simulink model "HQEV_MiL_20160830_integrate"  (Simulink 8.3)
settings: Solver=FixedStepDiscrete  StartTime=0.0  StopTime=inf  FixedStep=0.01  RelTol=1e-3
PostLoadFcn:
  | , if any(exist('dsrtsu_mdlpostloadfcn', 'file') == [2, 3, 6]), try dsrtsu_mdlpostloadfcn('Execute', bdroot); catch fprintf('Error in PostLoadFcn (dsrtsu_mdlpostloadfcn) for model "%s":\n %s\n', bdroot, lasterr); end, end,
values from neighbouring files (symbols this model uses):
  Bat_C_Ah = 36    [parameter_V1.mat]
  Bat_ocv_xIndex = [5 10 20 30 40 50 60 70 80 90 95]    [parameter_V1.mat]
  Bat_ocv_z = [329 332 340 345 347 351 358 372 377 386 391]    [parameter_V1.mat]
  Bat_R_ohm_z = [4.41 3.46 1.57 1.07 0.76 0.63 0.55 0.44 0.41 0.4 0.4 3.14 ... (66 elements, 11x6)]    [parameter_V1.mat]
  Bat_SOC_Init = 90    [parameter_V1.mat]
  Env_hum_pct_Ambient = 30    [parameter_V1.mat]
  Env_Slope_deg = 0    [parameter_V1.mat]
  Env_Temp_degC_Ambient = 25    [parameter_V1.mat]
  Env_v_kmph_HWind = 0    [parameter_V1.mat]
  Reducer_F_i = 7.23    [parameter_V1.mat]
  Reducer_R_i = 7.23    [parameter_V1.mat]
  Veh =     [parameter_V1.mat]
  Veh_A_m2_Fr = 2.246    [parameter_V1.mat]
  Veh_F_Brake =     [parameter_V1.mat]
  Veh_fac_AirDrag = 0.326    [parameter_V1.mat]
  Veh_fac_WhDragFrict_0 = 0.011    [parameter_V1.mat]
  Veh_g_mps2_C = 9.81    [parameter_V1.mat]
  Veh_GainBrake =     [parameter_V1.mat]
  Veh_h_m_COGHigh = 0.5    [parameter_V1.mat]
  Veh_J_kgm2_Wh = 1.3635    [parameter_V1.mat]
  Veh_L_m_AxlBas = 2.63    [parameter_V1.mat]
  Veh_M_kg = 1427    [parameter_V1.mat]
  Veh_mu_Brake = 0.4    [parameter_V1.mat]
  Veh_mu_Tyre =     [parameter_V1.mat]
  Veh_num_FrictPair = 8    [parameter_V1.mat]
  Veh_pct_Brk = 70    [parameter_V1.mat]
  Veh_r_dyn =     [parameter_V1.mat]
  Veh_r_m_BrkDisk = 0.136    [parameter_V1.mat]
  Veh_rho_kgpm3_Air = 1.2258    [parameter_V1.mat]
undefined symbols (not defined in the file or in its folder): DiscIntNeverNeededParam, p_bool_False_M, p_bool_True_M
libraries: BaseOperationLib_Browser x38, simulink x9, DTQC_lib x1, ERR_lib x1, MQM_lib x1, PTCL_lib x1, PUD_lib x1, TQD_lib x1, TQR_lib x1, VMM_lib x1, ACCA_lib x1, BBCA_lib x1
(part 13 of 15)

== system HQEV_MiL_20160830_integrate/MiL/Test_Integration/Charger/Charger/Charger/Charger/Abnormal/Subsystem ==
  Constant2 : Constant  Value=3
  Constant3 : Constant  Value=0
  Constant4 : Constant  Value=0
  Constant5 : Constant  Value=0
  Constant6 : Constant  Value=30
  ChargerOutputVoltage : Outport
  ChargerOutputCurrent : Outport  Port=2
  ChargerStatus : Outport  Port=3
  RechargeRequest : Outport  Port=4
  ChargerTemperature : Outport  Port=5
  wires:
  Constant2/1 -> ChargerStatus/1
  Constant5/1 -> RechargeRequest/1
  Constant6/1 -> ChargerTemperature/1
  Constant3/1 -> ChargerOutputVoltage/1
  Constant4/1 -> ChargerOutputCurrent/1

== system HQEV_MiL_20160830_integrate/MiL/Test_Integration/Charger/Charger/Charger/Charger/Fault/Subsystem ==
  Constant2 : Constant  Value=3
  Constant3 : Constant  Value=0
  Constant4 : Constant  Value=0
  Constant5 : Constant  Value=0
  Constant6 : Constant  Value=30
  ChargerOutputVoltage : Outport
  ChargerOutputCurrent : Outport  Port=2
  ChargerStatus : Outport  Port=3
  RechargeRequest : Outport  Port=4
  ChargerTemperature : Outport  Port=5
  wires:
  Constant2/1 -> ChargerStatus/1
  Constant5/1 -> RechargeRequest/1
  Constant6/1 -> ChargerTemperature/1
  Constant3/1 -> ChargerOutputVoltage/1
  Constant4/1 -> ChargerOutputCurrent/1

== system HQEV_MiL_20160830_integrate/MiL/Test_Integration/Charger/Charger/Charger/Charger/Idle/Subsystem ==
  CC : Inport
  ACChargeStation_U : Inport  Port=2
  Chart : Stateflow chart  TreatAsAtomicUnit=on
  Constant : Constant  Value=200
  Constant1 : Constant  Value=0
  Constant2 : Constant  Value=0
  Constant3 : Constant  Value=0
  Constant4 : Constant  Value=30
  Logical Operator : Logic  Operator=NOT  AllPortsSameDT=off  OutDataTypeStr=boolean
  Relational Operator : RelationalOperator  OutDataTypeStr=boolean
  ChargerOutputVoltage : Outport
  ChargerOutputCurrent : Outport  Port=2
  ChargerStatus : Outport  Port=3
  RechargeRequest : Outport  Port=4
  ChargerTemperature : Outport  Port=5
  wires:
  ACChargeStation_U/1 -> Relational Operator/1
  Constant/1 -> Relational Operator/2
  Relational Operator/1 -> Chart/1(PowerOn), Logical Operator/1
  Logical Operator/1 -> Chart/2(PowerOff)
  CC/1 -> Chart/3(CC)
  Chart/1(RechargeRequest) -> RechargeRequest/1
  Constant1/1 -> ChargerOutputVoltage/1
  Constant2/1 -> ChargerStatus/1
  Constant3/1 -> ChargerOutputCurrent/1
  Constant4/1 -> ChargerTemperature/1

== system HQEV_MiL_20160830_integrate/MiL/Test_Integration/Charger/Charger/Charger/Charger/Work/Subsystem ==
  HCU_ChargePermission : Inport
  BMS_MainPosContactorState : Inport  Port=2
  HCU_ChargeHeatingPermission : Inport  Port=3
  BMS_MainNegContactorState : Inport  Port=4
  BMS_PreChargeContactorState : Inport  Port=5
  BMS_ChargePosContactorState : Inport  Port=6
  BMS_ChargeNegContactorState : Inport  Port=7
  AC_Charge : Subsystem  TreatAsAtomicUnit=on
  Constant : Subsystem
  ChargerOutputVoltage : Outport
  ChargerOutputCurrent : Outport  Port=2
  ChargerStatus : Outport  Port=3
  RechargeRequest : Outport  Port=4
  ChargerTemperature : Outport  Port=5
  wires:
  AC_Charge/1(ChargerOutputVoltage) -> ChargerOutputVoltage/1
  AC_Charge/2(ChargerOutputCurrent) -> ChargerOutputCurrent/1
  Constant/1(ChargerStatus) -> ChargerStatus/1
  Constant/2(RechargeRequest) -> RechargeRequest/1
  Constant/3(ChargerTemperature) -> ChargerTemperature/1
  HCU_ChargePermission/1 -> AC_Charge/1(HCU_ChargePermission)
  BMS_MainPosContactorState/1 -> AC_Charge/2(BMS_MainPosContactorState)
  HCU_ChargeHeatingPermission/1 -> AC_Charge/3(HCU_ChargeHeatingPermission)
  BMS_MainNegContactorState/1 -> AC_Charge/4(BMS_MainNegContactorState)
  BMS_PreChargeContactorState/1 -> AC_Charge/5(BMS_PreChargeContactorState)
  BMS_ChargePosContactorState/1 -> AC_Charge/6(BMS_ChargePosContactorState)
  BMS_ChargeNegContactorState/1 -> AC_Charge/7(BMS_ChargeNegContactorState)

== system HQEV_MiL_20160830_integrate/MiL/Test_Integration/Driver/Driver/Driver_AutoPedal/CTRL AccPed/Reset/Compare To Constant ==
  u : Inport
  Compare : RelationalOperator  Operator=<  OutDataTypeStr=boolean  ZeroCross=off  InputSameDT=on
  Constant : Constant  Value=const  OutDataTypeStr=Inherit: Inherit via back propagation
  y : Outport
  wires:
  u/1 -> Compare/1
  Constant/1 -> Compare/2
  Compare/1 -> y/1

== system HQEV_MiL_20160830_integrate/MiL/Test_Integration/Driver/Driver/Driver_AutoPedal/CTRL AccPed/Reset/Compare To Constant1 ==
  u : Inport
  Compare : RelationalOperator  Operator=>  OutDataTypeStr=boolean  ZeroCross=off  InputSameDT=on
  Constant : Constant  Value=const  OutDataTypeStr=Inherit: Inherit via back propagation
  y : Outport
  wires:
  u/1 -> Compare/1
  Constant/1 -> Compare/2
  Compare/1 -> y/1

== system HQEV_MiL_20160830_integrate/MiL/Test_Integration/Driver/Driver/Driver_AutoPedal/CTRL AccPed/Reset/v_Set==0  ==
  u : Inport
  Compare : RelationalOperator  Operator=<=  OutDataTypeStr=uint(8)  ZeroCross=off  InputSameDT=on
  Constant : Constant  Value=const  OutDataTypeStr=Inherit: Inherit via back propagation
  y : Outport
  wires:
  u/1 -> Compare/1
  Constant/1 -> Compare/2
  Compare/1 -> y/1

== system HQEV_MiL_20160830_integrate/MiL/Test_Integration/Driver/Driver/Driver_AutoPedal/CTRL BrakePed/Reset_Block/Compare To Constant2 ==
  u : Inport
  Compare : RelationalOperator  Operator=>  OutDataTypeStr=uint(8)  ZeroCross=off  InputSameDT=on
  Constant : Constant  Value=const  OutDataTypeStr=Inherit: Inherit via back propagation
  y : Outport
  wires:
  Compare/1 -> y/1
  Constant/1 -> Compare/2
  u/1 -> Compare/1

== system HQEV_MiL_20160830_integrate/MiL/Test_Integration/Driver/Driver/Driver_AutoPedal/CTRL BrakePed/Reset_Block/Compare To Constant7 ==
  u : Inport
  Compare : RelationalOperator  Operator===  OutDataTypeStr=uint(8)  ZeroCross=off  InputSameDT=on
  Constant : Constant  Value=const  OutDataTypeStr=Inherit: Inherit via back propagation
  y : Outport
  wires:
  Compare/1 -> y/1
  Constant/1 -> Compare/2
  u/1 -> Compare/1

== system HQEV_MiL_20160830_integrate/MiL/Test_Integration/Driver/Driver/Driver_AutoPedal/CTRL BrakePed/Set_Block/Compare To Constant1 ==
  u : Inport
  Compare : RelationalOperator  Operator=<  OutDataTypeStr=boolean  ZeroCross=off  InputSameDT=on
  Constant : Constant  Value=const  OutDataTypeStr=Inherit: Inherit via back propagation
  y : Outport
  wires:
  Compare/1 -> y/1
  Constant/1 -> Compare/2
  u/1 -> Compare/1

== system HQEV_MiL_20160830_integrate/MiL/Test_Integration/Driver/Driver/Driver_AutoPedal/CTRL BrakePed/Set_Block/Compare To Constant3 ==
  u : Inport
  Compare : RelationalOperator  Operator=>  OutDataTypeStr=boolean  ZeroCross=off  InputSameDT=on
  Constant : Constant  Value=const  OutDataTypeStr=Inherit: Inherit via back propagation
  y : Outport
  wires:
  Compare/1 -> y/1
  Constant/1 -> Compare/2
  u/1 -> Compare/1

== system HQEV_MiL_20160830_integrate/MiL/Test_Integration/Driver/Driver/Driver_AutoPedal/CTRL BrakePed/Set_Block/Compare To Constant5 ==
  u : Inport
  Compare : RelationalOperator  Operator===  OutDataTypeStr=boolean  ZeroCross=off  InputSameDT=on
  Constant : Constant  Value=const  OutDataTypeStr=Inherit: Inherit via back propagation
  y : Outport
  wires:
  Compare/1 -> y/1
  Constant/1 -> Compare/2
  u/1 -> Compare/1

== system HQEV_MiL_20160830_integrate/MiL/Test_Integration/Driver/Driver/Driver_AutoPedal/CTRL BrakePed/Set_Block/Compare To Constant6 ==
  u : Inport
  Compare : RelationalOperator  Operator=>  OutDataTypeStr=boolean  ZeroCross=off  InputSameDT=on
  Constant : Constant  Value=const  OutDataTypeStr=Inherit: Inherit via back propagation
  y : Outport
  wires:
  Compare/1 -> y/1
  Constant/1 -> Compare/2
  u/1 -> Compare/1

== system HQEV_MiL_20160830_integrate/MiL/Test_Integration/Driver/Driver/Driver_AutoPedal/CTRL BrakePed/velocoty/Run_Forward ==
  v_set : Inport
  v_Veh : Inport  Port=2
  Difference : Subsystem
      mask Display: disp('')
  Gain1 : Gain  Gain=-1
  Subtract : Sum  Inputs=+-
  delta_v_set : Outport
  error : Outport  Port=2
  wires:
  v_set/1 -> Difference/1(In1), Subtract/1
  v_Veh/1 -> Subtract/2
  Difference/1(Out1) -> delta_v_set/1
  Subtract/1 -> Gain1/1
  Gain1/1 -> error/1

== system HQEV_MiL_20160830_integrate/MiL/Test_Integration/HCU/HCU/HCU/EVManager/evm_core/DTQC ==
  Bus_TQD : Inport
  Bus_hw_prep : Inport  Port=2
  Bus_hw_algo : Inport  Port=3
  Bus_PTC1 : BusSelector  OutputSignals=pTQD_Nm_MCU1TMTorqReq,pTQD_Nm_MCU2TMTorqReq
  Bus_PTC2 : BusSelector  OutputSignals=Bus_ESPI.pESPI_bool_ABSIntv,Bus_ESPI.pESPI_Nm_ABS1IntvTrqReq,Bus_ESPI.pESPI_Nm_ABS2IntvTrqReq,Bus_ESPI.pESPI_bool_ASR1Intv,Bus_ESPI.pESPI_Nm_ASR1IntvTrqReq,Bus_ESPI.pESPI_bool_ASR2Intv,Bus_ESPI.pESPI_Nm_ASR2IntvTrqReq,Bus_ESPI.pESPI_bool_RBSIntv,Bus_ESPI.pESPI_Nm_RBSIntvTrqReq,Bus_ESPI.pESPI_bool_MSR1Intv,Bus_ESPI.pESPI_Nm_MSR1IntvTrqReq,Bus_ESPI.pESPI_bool_MSR2Intv,Bus_ESPI.pESPI_Nm_MSR2IntvTrqReq
  Bus_PTC3 : BusSelector  OutputSignals=Bus_ACCI.pACCI_bool_AEBIntv,Bus_ACCI.pACCI_Nm_AEBTM1TrqReq,Bus_ACCI.pACCI_Nm_AEBTM2TrqReq
  Bus_TQD_out : BusCreator  Inputs=3
  DTQC : DTQC_lib/DTQC  SystemSampleTime=-1
  Terminator : Terminator
  Bus_DTQC : Outport
  wires:
  Bus_PTC3/3 -> DTQC/18  "<pACCI_Nm_AEBTM2TrqReq>"
  Bus_PTC3/2 -> DTQC/17  "<pACCI_Nm_AEBTM1TrqReq>"
  Bus_PTC3/1 -> DTQC/16  "<pACCI_bool_AEBIntv>"
  Bus_hw_algo/1 -> Terminator/1
  Bus_PTC2/13 -> DTQC/13  "<pESPI_Nm_MSR2IntvTrqReq>"
  Bus_PTC2/12 -> DTQC/12  "<pESPI_bool_MSR2Intv>"
  Bus_PTC2/11 -> DTQC/11  "<pESPI_Nm_MSR1IntvTrqReq>"
  Bus_PTC2/10 -> DTQC/10  "<pESPI_bool_MSR1Intv>"
  Bus_PTC2/9 -> DTQC/9  "<pESPI_Nm_RBSIntvTrqReq>"
  Bus_PTC2/8 -> DTQC/8  "<pESPI_bool_RBSIntv>"
  Bus_PTC2/7 -> DTQC/7  "<pESPI_Nm_ASR2IntvTrqReq>"
  Bus_PTC2/6 -> DTQC/6  "<pESPI_bool_ASR2Intv>"
  Bus_PTC2/5 -> DTQC/5  "<pESPI_Nm_ASR1IntvTrqReq>"
  Bus_PTC2/4 -> DTQC/4  "<pESPI_bool_ASR1Intv>"
  Bus_PTC2/3 -> DTQC/3  "<pESPI_Nm_ABS2IntvTrqReq>"
  Bus_PTC2/2 -> DTQC/2  "<pESPI_Nm_ABS1IntvTrqReq>"
  Bus_PTC2/1 -> DTQC/1  "<pESPI_bool_ABSIntv>"
  Bus_hw_prep/1 -> Bus_PTC3/1, Bus_PTC2/1
  Bus_PTC1/2 -> DTQC/15  "<pTQD_Nm_MCU2TMTorqReq>"
  Bus_PTC1/1 -> DTQC/14  "<pTQD_Nm_MCU1TMTorqReq>"
  DTQC/3 -> Bus_TQD_out/3
  DTQC/2 -> Bus_TQD_out/2
  DTQC/1 -> Bus_TQD_out/1
  Bus_TQD/1 -> Bus_PTC1/1
  Bus_TQD_out/1 -> Bus_DTQC/1  "Bus_DTQC"

== system HQEV_MiL_20160830_integrate/MiL/Test_Integration/HCU/HCU/HCU/EVManager/evm_core/ERR ==
  Bus_hw_prep : Inport
  Bus_hw_algo : Inport  Port=2
  Bus Selector : BusSelector  OutputSignals=Bus_ARBI.pARBI_st_StCrash,Bus_MCI.pMCI_st_MotCtrlErr,Bus_TBCI.pTBCI_st_ChrgrErr,Bus_BMSI.pBMSI_st_BMSErr,Bus_SHLI.pSHLI_st_ShftLvrErr,Bus_ESPI.pESPI_kmph_VehLgtSpd
  Bus Selector1 : BusSelector  OutputSignals=Bus_SHLA.pSHLA_st_PrkgLockFlt
  Bus Selector2 : BusSelector  OutputSignals=Bus_BRPI.pBRPI_st_BrkPedErr,Bus_ARBI.pARBI_st_AirBagErr,Bus_EPSI.pEPSI_st_EPSErr,Bus_DCCI.pDCCI_st_DCDCErr,Bus_TMCI.pTMCI_bool_AirCdnErr,Bus_TMCI.pTMCI_st_AC1PTCSt
  Bus Selector4 : BusSelector  OutputSignals=Bus_TBCI.pTBCI_st_ChrgrPlgTempErr,Bus_BMSI.pBMSI_st_DCChrgrErr
  ERR : ERR_lib/ERR  SystemSampleTime=-1
  err_bb : BusCreator  Inputs=2
  Bus_ERR : Outport
  wires:
  Bus Selector/6 -> ERR/6  "<pESPI_kmph_VehLgtSpd>"
  ERR/2 -> err_bb/2
  Bus Selector2/2 -> ERR/9  "<pARBI_st_AirBagErr>"
  Bus Selector2/1 -> ERR/8  "<pBRPI_st_BrkPedErr>"
  Bus Selector4/2 -> ERR/15  "<pBMSI_st_DCChrgrErr>"
  Bus Selector4/1 -> ERR/14  "<pTBCI_st_ChrgrPlgTempErr>"
  Bus Selector2/5 -> ERR/12  "<pTMCI_bool_AirCdnErr>"
  Bus Selector2/4 -> ERR/11  "<pDCCI_st_DCDCErr>"
  Bus Selector2/3 -> ERR/10  "<pEPSI_st_EPSErr>"
  Bus Selector1/1 -> ERR/7  "<pSHLA_st_PrkgLockFlt>"
  Bus_hw_algo/1 -> Bus Selector1/1
  Bus Selector/5 -> ERR/5  "<pSHLI_st_ShftLvrErr>"
  Bus Selector/4 -> ERR/4  "<pBMSI_st_BMSErr>"
  Bus Selector/3 -> ERR/3  "<pTBCI_st_ChrgrErr>"
  Bus Selector/2 -> ERR/2  "<pMCI_st_MotCtrlErr>"
  Bus Selector/1 -> ERR/1  "<pARBI_st_StCrash>"
  ERR/1 -> err_bb/1
  err_bb/1 -> Bus_ERR/1  "Bus_ERR"
  Bus_hw_prep/1 -> Bus Selector/1, Bus Selector4/1, Bus Selector2/1
  Bus Selector2/6 -> ERR/13  "<pTMCI_st_AC1PTCSt>"

== system HQEV_MiL_20160830_integrate/MiL/Test_Integration/HCU/HCU/HCU/EVManager/evm_core/MQM ==
  Bus_DTQC : Inport
  Bus_hw_prep : Inport  Port=2
  Bus_hw_algo : Inport  Port=3
  Bus_PTC1 : BusSelector  OutputSignals=pDTQC_Nm_MCU1TMTorqReq,pDTQC_Nm_MCU2TMTorqReq
  Bus_PTC2 : BusSelector  OutputSignals=Bus_MCI.pMCI_Nm_MCU1MotCtrlActTrq,Bus_MCI.pMCI_Nm_MCU2MotCtrlActTrq
  Bus_PTC3 : BusSelector  OutputSignals=Bus_SHLA.pSHLA_st_ShiftLvrPosn
  Bus_TQD_out : BusCreator  Inputs=3
  MQM : MQM_lib/MQM  SystemSampleTime=-1
  Bus_MQM : Outport
  wires:
  Bus_PTC3/1 -> MQM/5  "<pSHLA_st_ShiftLvrPosn>"
  Bus_hw_algo/1 -> Bus_PTC3/1
  Bus_PTC2/2 -> MQM/4  "<pMCI_Nm_MCU2MotCtrlActTrq>"
  Bus_PTC2/1 -> MQM/3  "<pMCI_Nm_MCU1MotCtrlActTrq>"
  Bus_hw_prep/1 -> Bus_PTC2/1
  Bus_PTC1/2 -> MQM/2  "<pDTQC_Nm_MCU2TMTorqReq>"
  Bus_PTC1/1 -> MQM/1  "<pDTQC_Nm_MCU1TMTorqReq>"
  Bus_TQD_out/1 -> Bus_MQM/1  "Bus_MQM"
  Bus_DTQC/1 -> Bus_PTC1/1
  MQM/1 -> Bus_TQD_out/1
  MQM/2 -> Bus_TQD_out/2
  MQM/3 -> Bus_TQD_out/3

== system HQEV_MiL_20160830_integrate/MiL/Test_Integration/HCU/HCU/HCU/EVManager/evm_core/PTCL ==
  Bus_hw_prep : Inport
  PTCL : PTCL_lib/PTCL  SystemSampleTime=-1
  egc_bb : BusCreator  Inputs=12
  hwprep_egc : BusSelector  OutputSignals=Bus_BMSI.pBMSI_kw_ChrgPwrAvail10,Bus_BMSI.pBMSI_kw_DischrgPwrAvail10,Bus_BMSI.pBMSI_kw_ChrgPwrAvail2,Bus_BMSI.pBMSI_kw_DischrgPwrAvail2,Bus_BMSI.pBMSI_V_BatActVolt,Bus_TMCI.pTMCI_w_AC1PwrCnsmpACHi,Bus_BMSI.pBMSI_A_BatActCurr,Bus_DCCI.pDCCI_A_DCDCActInpCurr,Bus_MCI.pMCI_rpm_MCU1MotCtrlActRev,Bus_MCI.pMCI_rpm_MCU2MotCtrlActRev,Bus_ESPI.pESPI_kmph_VehLgtSpd,Bus_MCI.pMCI_Nm_MCU1DrvTrqLim,Bus_MCI.pMCI_Nm_MCU1RcpTrqLim,Bus_MCI.pMCI_pct_MCU1MotDrvEffi,Bus_MCI.pMCI_pct_MCU1MotRcpEffi,Bus_MCI.pMCI_Nm_MCU2DrvTrqLim,Bus_MCI.pMCI_Nm_MCU2RcpTrqLim,Bus_MCI.pMCI_pct_MCU2MotDrvEffi,Bus_MCI.pMCI_pct_MCU2MotRcpEffi
  Bus_PTCL : Outport
  wires:
  PTCL/12 -> egc_bb/12
  PTCL/11 -> egc_bb/11
  PTCL/10 -> egc_bb/10
  PTCL/9 -> egc_bb/9
  PTCL/8 -> egc_bb/8
  PTCL/7 -> egc_bb/7
  PTCL/6 -> egc_bb/6
  PTCL/5 -> egc_bb/5
  PTCL/4 -> egc_bb/4
  PTCL/3 -> egc_bb/3
  PTCL/2 -> egc_bb/2
  PTCL/1 -> egc_bb/1
  hwprep_egc/19 -> PTCL/19  "<pMCI_pct_MCU2MotRcpEffi>"
  hwprep_egc/18 -> PTCL/18  "<pMCI_pct_MCU2MotDrvEffi>"
  hwprep_egc/17 -> PTCL/17  "<pMCI_Nm_MCU2RcpTrqLim>"
  hwprep_egc/16 -> PTCL/16  "<pMCI_Nm_MCU2DrvTrqLim>"
  hwprep_egc/15 -> PTCL/15  "<pMCI_pct_MCU1MotRcpEffi>"
  hwprep_egc/14 -> PTCL/14  "<pMCI_pct_MCU1MotDrvEffi>"
  hwprep_egc/13 -> PTCL/13  "<pMCI_Nm_MCU1RcpTrqLim>"
  hwprep_egc/12 -> PTCL/12  "<pMCI_Nm_MCU1DrvTrqLim>"
  hwprep_egc/11 -> PTCL/11  "<pESPI_kmph_VehLgtSpd>"
  hwprep_egc/10 -> PTCL/10  "<pMCI_rpm_MCU2MotCtrlActRev>"
  hwprep_egc/9 -> PTCL/9  "<pMCI_rpm_MCU1MotCtrlActRev>"
  hwprep_egc/8 -> PTCL/8  "<pDCCI_A_DCDCActInpCurr>"
  hwprep_egc/7 -> PTCL/7  "<pBMSI_A_BatActCurr>"
  hwprep_egc/6 -> PTCL/6  "<pTMCI_w_AC1PwrCnsmpACHi>"
  hwprep_egc/5 -> PTCL/5  "<pBMSI_V_BatActVolt>"
  hwprep_egc/4 -> PTCL/4  "<pBMSI_kw_DischrgPwrAvail2>"
  hwprep_egc/3 -> PTCL/3  "<pBMSI_kw_ChrgPwrAvail2>"
  hwprep_egc/2 -> PTCL/2  "<pBMSI_kw_DischrgPwrAvail10>"
  hwprep_egc/1 -> PTCL/1  "<pBMSI_kw_ChrgPwrAvail10>"
  egc_bb/1 -> Bus_PTCL/1  "Bus_PTCL"
  Bus_hw_prep/1 -> hwprep_egc/1

== system HQEV_MiL_20160830_integrate/MiL/Test_Integration/HCU/HCU/HCU/EVManager/evm_core/PUD ==
  Bus_hw_prep : Inport
  Bus_hw_algo : Inport  Port=2
  Bus_VMM : Inport  Port=3
  Constant : BaseOperationLib_Browser/Sources&Sinks/Constant  Value=0  OutMin=[]  OutMax=[]  OutDataTypeMode=uint32  OutDataType=fixdt(1, 16)  ConRadixGroup=Use specified scaling  OutScaling=2^0  OutDataTypeStr=uint32
  PUD : PUD_lib/PUD  SystemSampleTime=-1
  egc_bb : BusCreator  Inputs=12
  hwprep_egc : BusSelector  OutputSignals=Bus_MCI.pMCI_bool_MCU1ShtdwnAllow,Bus_MCI.pMCI_bool_MCU2ShtdwnAllow,Bus_MCI.pMCI_V_MCU1MotCapVolt,Bus_MCI.pMCI_V_MCU2MotCapVolt,Bus_TBCI.pTBCI_bool_ACChrgrPlugDtctd,Bus_TBCI.pTBCI_bool_DCChrgrPlugDtctd
  hwprep_egc6 : BusSelector  OutputSignals=signal6.pTMCA_bool_HvPwrOffEnbl,Bus_BMSA.pBMSA_st_BmsSt,Bus_TBCA.pTBCA_st_ChrgrSts,Bus_DCCA.pDCCA_st_DcDcActSts
  ptc_eg_bs : BusSelector  OutputSignals=pVMM_st_PUDCoorrReq
  Bus_PUD : Outport
  wires:
  Constant/1 -> PUD/12
  PUD/12 -> egc_bb/12
  hwprep_egc/4 -> PUD/5  "<pMCI_V_MCU2MotCapVolt>"
  hwprep_egc/3 -> PUD/4  "<pMCI_V_MCU1MotCapVolt>"
  PUD/11 -> egc_bb/11
  PUD/10 -> egc_bb/10
  PUD/9 -> egc_bb/9
  PUD/8 -> egc_bb/8
  PUD/7 -> egc_bb/7
  PUD/6 -> egc_bb/6
  hwprep_egc6/1 -> PUD/8  "<pTMCA_bool_HvPwrOffEnbl>"
  hwprep_egc6/2 -> PUD/9  "<pBMSA_st_BmsSt>"
  hwprep_egc6/3 -> PUD/10  "<pTBCA_st_ChrgrSts>"
  PUD/5 -> egc_bb/5
  PUD/4 -> egc_bb/4
  PUD/3 -> egc_bb/3
  PUD/2 -> egc_bb/2
  PUD/1 -> egc_bb/1
  hwprep_egc/2 -> PUD/3  "<pMCI_bool_MCU2ShtdwnAllow>"
  hwprep_egc/1 -> PUD/2  "<pMCI_bool_MCU1ShtdwnAllow>"
  egc_bb/1 -> Bus_PUD/1  "Bus_PUD"
  Bus_VMM/1 -> ptc_eg_bs/1
  Bus_hw_prep/1 -> hwprep_egc/1
  ptc_eg_bs/1 -> PUD/1  "<pVMM_st_PUDCoorrReq>"
  Bus_hw_algo/1 -> hwprep_egc6/1
  hwprep_egc6/4 -> PUD/11  "<pDCCA_st_DcDcActSts>"
  hwprep_egc/5 -> PUD/6  "<pTBCI_bool_ACChrgrPlugDtctd>"
  hwprep_egc/6 -> PUD/7  "<pTBCI_bool_DCChrgrPlugDtctd>"

== system HQEV_MiL_20160830_integrate/MiL/Test_Integration/HCU/HCU/HCU/EVManager/evm_core/TQD ==
  Bus_TQR : Inport
  Bus_hw_prep : Inport  Port=2
  Bus_hw_algo : Inport  Port=3
  Bus_PTC1 : BusSelector  OutputSignals=pTQR_Nm_DrvrTqReq
  Bus_PTC2 : BusSelector  OutputSignals=Bus_MCI.pMCI_Nm_MCU1MotCtrlActTrq,Bus_MCI.pMCI_Nm_MCU2MotCtrlActTrq
  Bus_PTC4 : BusSelector  OutputSignals=Bus_MCI.pMCI_rpm_MCU1MotCtrlActRev,Bus_MCI.pMCI_rpm_MCU2MotCtrlActRev
  Bus_TQD_out : BusCreator  Inputs=3
  TQD : TQD_lib/TQD  SystemSampleTime=-1
  Terminator : Terminator
  Bus_TQD : Outport
  wires:
  Bus_hw_algo/1 -> Terminator/1
  Bus_PTC4/2 -> TQD/5  "<pMCI_rpm_MCU2MotCtrlActRev>"
  Bus_PTC4/1 -> TQD/4  "<pMCI_rpm_MCU1MotCtrlActRev>"
  TQD/1 -> Bus_TQD_out/1
  TQD/2 -> Bus_TQD_out/2
  TQD/3 -> Bus_TQD_out/3
  Bus_TQD_out/1 -> Bus_TQD/1  "Bus_TQD"
  Bus_TQR/1 -> Bus_PTC1/1
  Bus_PTC1/1 -> TQD/1  "<pTQR_Nm_DrvrTqReq>"
  Bus_hw_prep/1 -> Bus_PTC4/1, Bus_PTC2/1
  Bus_PTC2/1 -> TQD/2  "<pMCI_Nm_MCU1MotCtrlActTrq>"
  Bus_PTC2/2 -> TQD/3  "<pMCI_Nm_MCU2MotCtrlActTrq>"

== system HQEV_MiL_20160830_integrate/MiL/Test_Integration/HCU/HCU/HCU/EVManager/evm_core/TQR ==
  Bus_PTCL : Inport
  Bus_hw_prep : Inport  Port=2
  Bus_hw_algo : Inport  Port=3
  Bus Selector1 : BusSelector  OutputSignals=Bus_ACPI.pACPI_pct_AccPedVal,Bus_SHLI.pSHLI_st_ECOSwtSt,Bus_BRPI.pBRPI_bool_BrkPedPrsd,Bus_BRPI.pBRPI_bar_BrkPedPres
  Bus Selector3 : BusSelector  OutputSignals=Bus_SHLA.pSHLA_st_ShiftLvrPosn
  TQR : TQR_lib/TQR  SystemSampleTime=-1
  bus_TQR : BusCreator  Inputs=3
  err_bs1 : BusSelector  OutputSignals=pPTCL_Nm_MotContiDrvTrqLim,pPTCL_Nm_MotContiRcpTrqLim
  err_bs4 : BusSelector  OutputSignals=Bus_ESPI.pESPI_kmph_VehLgtSpd
  err_bs6 : BusSelector  OutputSignals=Bus_MCI.pMCI_rpm_MCU1MotCtrlActRev,Bus_MCI.pMCI_rpm_MCU2MotCtrlActRev,Bus_MCI.pMCI_Nm_MCU2MotCtrlActTrq,Bus_ACCI.pACCI_bool_ACCIntv,Bus_ACCI.pACCI_Nm_ACCTrqReq
  Bus_TQR : Outport
  wires:
  err_bs6/5 -> TQR/13  "<pACCI_Nm_ACCTrqReq>"
  err_bs6/4 -> TQR/12  "<pACCI_bool_ACCIntv>"
  err_bs6/3 -> TQR/11  "<pMCI_Nm_MCU2MotCtrlActTrq>"
  err_bs6/2 -> TQR/10  "<pMCI_rpm_MCU2MotCtrlActRev>"
  err_bs6/1 -> TQR/9  "<pMCI_rpm_MCU1MotCtrlActRev>"
  err_bs1/2 -> TQR/8  "<pPTCL_Nm_MotContiRcpTrqLim>"
  err_bs1/1 -> TQR/7  "<pPTCL_Nm_MotContiDrvTrqLim>"
  err_bs4/1 -> TQR/6  "<pESPI_kmph_VehLgtSpd>"
  Bus Selector3/1 -> TQR/5  "<pSHLA_st_ShiftLvrPosn>"
  Bus Selector1/4 -> TQR/4  "<pBRPI_bar_BrkPedPres>"
  Bus Selector1/3 -> TQR/3  "<pBRPI_bool_BrkPedPrsd>"
  Bus Selector1/2 -> TQR/2  "<pSHLI_st_ECOSwtSt>"
  Bus Selector1/1 -> TQR/1  "<pACPI_pct_AccPedVal>"
  Bus_hw_algo/1 -> Bus Selector3/1
  bus_TQR/1 -> Bus_TQR/1  "Bus_TQR"
  Bus_hw_prep/1 -> err_bs4/1, err_bs6/1, Bus Selector1/1
  TQR/1 -> bus_TQR/1
  TQR/2 -> bus_TQR/2
  TQR/3 -> bus_TQR/3
  Bus_PTCL/1 -> err_bs1/1

== system HQEV_MiL_20160830_integrate/MiL/Test_Integration/HCU/HCU/HCU/EVManager/evm_core/VMM ==
  Bus_hw_prep : Inport
  Bus_hw_algo : Inport  Port=2
  Bus_PUD : Inport  Port=3
  Bus_ERR : Inport  Port=4
  VMM : VMM_lib/VMM  SystemSampleTime=-1
  bus_subsystem_in : BusCreator
  hwalgo_ptc : BusSelector  OutputSignals=Bus_IGSI.pIGSI_st_OprtMode,Bus_IGSI.pIGSI_bool_Immo,Bus_SHLI.pSHLI_st_Epark,Bus_BMSI.pBMSI_bool_BatChrgReq,Bus_BMSI.pBMSI_bool_BatHeatReq,Bus_TBCI.pTBCI_bool_ACChrgrPlugDtctd,Bus_TBCI.pTBCI_bool_DCChrgrPlugDtctd,Bus_TBCI.pTBCI_bool_ReChrgReq,Bus_MCI.pMCI_bool_MCU1PrechrgAllow,Bus_MCI.pMCI_bool_MCU2PreChrgAllow,Bus_ESPI.pESPI_kmph_VehLgtSpd,Bus_BRPI.pBRPI_bool_BrkPedPrsd
  hwalgo_ptc1 : BusSelector  OutputSignals=pERR_st_ReactPTC
  hwalgo_ptc3 : BusSelector  OutputSignals=Bus_SHLA.pSHLA_st_ShiftLvrPosn,Bus_TBCA.pTBCA_bool_ChrgrCmpl,Bus_TBCA.pTBCA_bool_ChrgrHeatCmpl,signal6.pTMCA_bool_ShtdwnAck
  hwprep_ptc1 : BusSelector  OutputSignals=pPUD_st_CoorrSts,pPUD_st_AcChrgModeSt,pPUD_st_DcChrgModeSt,pPUD_st_AcHeatModeSt,pPUD_st_DcHeatModeSt,pPUD_st_HVOnModeSt
  Bus_VMM : Outport
  wires:
  hwalgo_ptc/12 -> VMM/12  "<pBRPI_bool_BrkPedPrsd>"
  hwalgo_ptc/11 -> VMM/11  "<pESPI_kmph_VehLgtSpd>"
  hwalgo_ptc/10 -> VMM/10  "<pMCI_bool_MCU2PreChrgAllow>"
  hwalgo_ptc/9 -> VMM/9  "<pMCI_bool_MCU1PrechrgAllow>"
  hwalgo_ptc/8 -> VMM/8  "<pTBCI_bool_ReChrgReq>"
  hwalgo_ptc/7 -> VMM/7  "<pTBCI_bool_DCChrgrPlugDtctd>"
  hwalgo_ptc/6 -> VMM/6  "<pTBCI_bool_ACChrgrPlugDtctd>"
  hwalgo_ptc/5 -> VMM/5  "<pBMSI_bool_BatHeatReq>"
  hwalgo_ptc/4 -> VMM/4  "<pBMSI_bool_BatChrgReq>"
  hwalgo_ptc/3 -> VMM/3  "<pSHLI_st_Epark>"
  hwalgo_ptc/2 -> VMM/2  "<pIGSI_bool_Immo>"
  hwalgo_ptc/1 -> VMM/1  "<pIGSI_st_OprtMode>"
  hwalgo_ptc3/3 -> VMM/15  "<pTBCA_bool_ChrgrHeatCmpl>"
  Bus_ERR/1 -> hwalgo_ptc1/1
  VMM/4 -> bus_subsystem_in/4
  VMM/3 -> bus_subsystem_in/3
  VMM/2 -> bus_subsystem_in/2
  VMM/1 -> bus_subsystem_in/1
  hwalgo_ptc1/1 -> VMM/23  "<pERR_st_ReactPTC>"
  hwprep_ptc1/6 -> VMM/22  "<pPUD_st_HVOnModeSt>"
  hwprep_ptc1/5 -> VMM/21  "<pPUD_st_DcHeatModeSt>"
  hwprep_ptc1/4 -> VMM/20  "<pPUD_st_AcHeatModeSt>"
  hwprep_ptc1/3 -> VMM/19  "<pPUD_st_DcChrgModeSt>"
  hwprep_ptc1/2 -> VMM/18  "<pPUD_st_AcChrgModeSt>"
  hwprep_ptc1/1 -> VMM/17  "<pPUD_st_CoorrSts>"
  hwalgo_ptc3/4 -> VMM/16  "<pTMCA_bool_ShtdwnAck>"
  hwalgo_ptc3/2 -> VMM/14  "<pTBCA_bool_ChrgrCmpl>"
  hwalgo_ptc3/1 -> VMM/13  "<pSHLA_st_ShiftLvrPosn>"
  Bus_PUD/1 -> hwprep_ptc1/1
  Bus_hw_prep/1 -> hwalgo_ptc/1
  Bus_hw_algo/1 -> hwalgo_ptc3/1
  bus_subsystem_in/1 -> Bus_VMM/1  "Bus_VMM"

== system HQEV_MiL_20160830_integrate/MiL/Test_Integration/MCU_FF/MCU/MCU/Rapid_Discharge/Subsystem/Subsystem ==
  EM_spd : Inport
  Constant : Constant  Value=170
  Constant1 : Constant  Value=0
  Constant2 : Constant
  Relational Operator : RelationalOperator  Operator=<  OutDataTypeStr=boolean
  Switch : Switch  Criteria=u2 ~= 0
  PWM : Outport
  wires:
  EM_spd/1 -> Relational Operator/1
  Constant/1 -> Relational Operator/2
  Relational Operator/1 -> Switch/2
  Constant1/1 -> Switch/1
  Constant2/1 -> Switch/3
  Switch/1 -> PWM/1

== system HQEV_MiL_20160830_integrate/MiL/Test_Integration/MCU_FF/MCU/MCU/Standby/Subsystem/Subsystem ==
  EM_spd : Inport
  Constant : Constant  Value=170
  Constant1 : Constant  Value=0
  Constant2 : Constant
  Relational Operator : RelationalOperator  Operator=<  OutDataTypeStr=boolean
  Switch : Switch  Criteria=u2 ~= 0
  PWM : Outport
  wires:
  EM_spd/1 -> Relational Operator/1
  Constant/1 -> Relational Operator/2
  Relational Operator/1 -> Switch/2
  Constant1/1 -> Switch/1
  Constant2/1 -> Switch/3
  Switch/1 -> PWM/1

== system HQEV_MiL_20160830_integrate/MiL/Test_Integration/MCU_FF/MCU/MCU/Stop/Subsystem/Subsystem ==
  EM_spd : Inport
  Constant : Constant  Value=170
  Constant1 : Constant  Value=0
  Constant2 : Constant
  Relational Operator : RelationalOperator  Operator=<  OutDataTypeStr=boolean
  Switch : Switch  Criteria=u2 ~= 0
  PWM : Outport
  wires:
  EM_spd/1 -> Relational Operator/1
  Constant/1 -> Relational Operator/2
  Relational Operator/1 -> Switch/2
  Constant1/1 -> Switch/1
  Constant2/1 -> Switch/3
  Switch/1 -> PWM/1

== system HQEV_MiL_20160830_integrate/MiL/Test_Integration/MCU_FF/MCU/MCU/Torque_Control/Subsystem/Max_Torque ==
  EM_Volt : Inport
  EM_spd : Inport  Port=2
  Max_Gen_Torque_Subsystem : Subsystem
  Max_Mot_Torque_Subsystem : Subsystem
  Unit Delay : UnitDelay  SampleTime=-1
  Unit Delay1 : UnitDelay  SampleTime=-1
  Max_Mot_Torque : Outport
  Max_Gen_Torque : Outport  Port=2
  wires:
  EM_spd/1 -> Max_Mot_Torque_Subsystem/2(EM_spd), Max_Gen_Torque_Subsystem/2(EM_spd)
  Max_Mot_Torque_Subsystem/1(Out1) -> Unit Delay/1
  EM_Volt/1 -> Max_Mot_Torque_Subsystem/1(EM_Volt), Max_Gen_Torque_Subsystem/1(EM_Volt)
  Max_Gen_Torque_Subsystem/1(Out1) -> Unit Delay1/1
  Unit Delay/1 -> Max_Mot_Torque/1
  Unit Delay1/1 -> Max_Gen_Torque/1

== system HQEV_MiL_20160830_integrate/MiL/Test_Integration/MCU_RR/MCU/MCU/Subsystem14/GSD/Subsystem ==
  In1 : Inport
  Constant11 : Constant
  Constant2 : Constant  Value=5
  Ground{,1..4,6..12} (12 alike) : Ground
  Terminator : Terminator
  MCU1_TMSpeed : Outport
  MCU1_ActTMTorque : Outport  Port=2
  MCU1_TMCapacitanceVoltage : Outport  Port=3
  MCU1_ActualTMTorqueValid : Outport  Port=4
  MCU1_MCU1 PrechargeAllow : Outport  Port=5
  MCU1_TMStatus : Outport  Port=6
  MCU1_TMErrorStatus : Outport  Port=7
  MCU1_TM MAMTorque : Outport  Port=8
  MCU1_TM MAGTorque : Outport  Port=9
  MCU1_CalTMTorque : Outport  Port=10
  MCU1_CoolingRequest : Outport  Port=11
  PWM_Status : Outport  Port=12
  EM_trq_req : Outport  Port=13
  bool_MCUPwrDwnAllow : Outport  Port=14
  wires:
  Ground/1 -> MCU1_TMSpeed/1
  Ground1/1 -> MCU1_ActTMTorque/1
  Ground2/1 -> MCU1_TMCapacitanceVoltage/1
  Ground3/1 -> MCU1_ActualTMTorqueValid/1
  Ground4/1 -> MCU1_MCU1 PrechargeAllow/1
  Constant2/1 -> MCU1_TMStatus/1
  Ground6/1 -> MCU1_TMErrorStatus/1
  Ground7/1 -> MCU1_TM MAMTorque/1
  Ground8/1 -> MCU1_TM MAGTorque/1
  Ground9/1 -> MCU1_CalTMTorque/1
  Ground10/1 -> MCU1_CoolingRequest/1
  Ground11/1 -> PWM_Status/1
  Ground12/1 -> EM_trq_req/1
  In1/1 -> Terminator/1
  Constant11/1 -> bool_MCUPwrDwnAllow/1

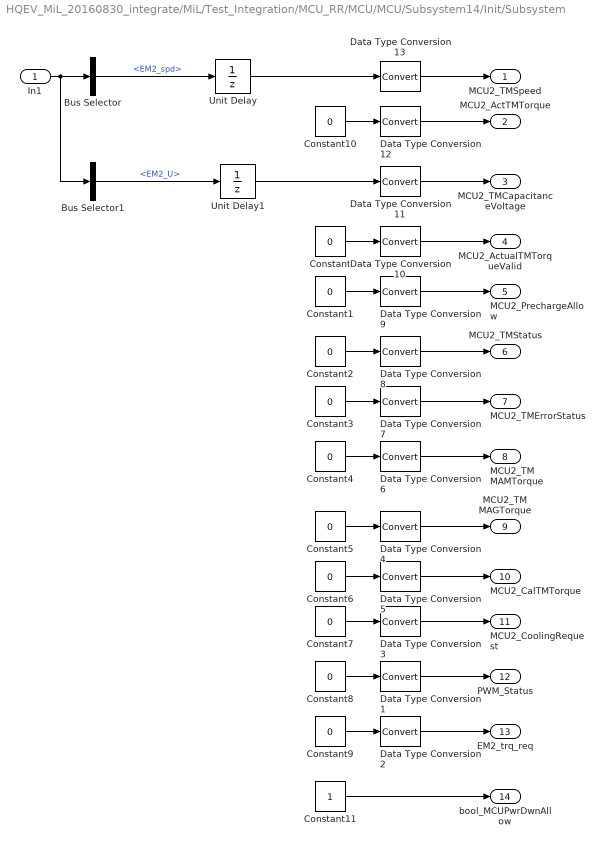
== system HQEV_MiL_20160830_integrate/MiL/Test_Integration/MCU_RR/MCU/MCU/Subsystem14/Init/Subsystem ==
  In1 : Inport
  Bus Selector : BusSelector  OutputSignals=Motor_R.EM2_spd
  Bus Selector1 : BusSelector  OutputSignals=Motor_R.EM2_U
  Constant{,1..10} (11 alike) : Constant  Value=0
  Constant11 : Constant
  Data Type Conversion{1..13} (13 alike) : DataTypeConversion
  Unit Delay : UnitDelay  SampleTime=-1
  Unit Delay1 : UnitDelay  SampleTime=-1
  MCU2_TMSpeed : Outport
  MCU2_ActTMTorque : Outport  Port=2
  MCU2_TMCapacitanceVoltage : Outport  Port=3
  MCU2_ActualTMTorqueValid : Outport  Port=4
  MCU2_PrechargeAllow : Outport  Port=5
  MCU2_TMStatus : Outport  Port=6
  MCU2_TMErrorStatus : Outport  Port=7
  MCU2_TM MAMTorque : Outport  Port=8
  MCU2_TM MAGTorque : Outport  Port=9
  MCU2_CalTMTorque : Outport  Port=10
  MCU2_CoolingRequest : Outport  Port=11
  PWM_Status : Outport  Port=12
  EM2_trq_req : Outport  Port=13
  bool_MCUPwrDwnAllow : Outport  Port=14
  wires:
  Constant/1 -> Data Type Conversion10/1
  Constant1/1 -> Data Type Conversion9/1
  Constant2/1 -> Data Type Conversion8/1
  Constant3/1 -> Data Type Conversion7/1
  Constant4/1 -> Data Type Conversion6/1
  Constant5/1 -> Data Type Conversion4/1
  Constant6/1 -> Data Type Conversion5/1
  Constant7/1 -> Data Type Conversion3/1
  Constant8/1 -> Data Type Conversion1/1
  Constant9/1 -> Data Type Conversion2/1
  Constant10/1 -> Data Type Conversion12/1
  In1/1 -> Bus Selector/1, Bus Selector1/1
  Bus Selector/1 -> Unit Delay/1  "<EM2_spd>"
  Bus Selector1/1 -> Unit Delay1/1  "<EM2_U>"
  Unit Delay/1 -> Data Type Conversion13/1
  Unit Delay1/1 -> Data Type Conversion11/1
  Data Type Conversion2/1 -> EM2_trq_req/1
  Data Type Conversion1/1 -> PWM_Status/1
  Data Type Conversion3/1 -> MCU2_CoolingRequest/1
  Data Type Conversion5/1 -> MCU2_CalTMTorque/1
  Data Type Conversion4/1 -> MCU2_TM MAGTorque/1
  Data Type Conversion6/1 -> MCU2_TM MAMTorque/1
  Data Type Conversion7/1 -> MCU2_TMErrorStatus/1
  Data Type Conversion8/1 -> MCU2_TMStatus/1
  Data Type Conversion9/1 -> MCU2_PrechargeAllow/1
  Data Type Conversion10/1 -> MCU2_ActualTMTorqueValid/1
  Data Type Conversion11/1 -> MCU2_TMCapacitanceVoltage/1
  Data Type Conversion12/1 -> MCU2_ActTMTorque/1
  Data Type Conversion13/1 -> MCU2_TMSpeed/1
  Constant11/1 -> bool_MCUPwrDwnAllow/1

== system HQEV_MiL_20160830_integrate/MiL/Test_Integration/MCU_RR/MCU/MCU/Subsystem14/Invalid/Subsystem ==
  In1 : Inport
  Constant11 : Constant
  Ground{,1..12} (13 alike) : Ground
  Terminator : Terminator
  MCU1_TMSpeed : Outport
  MCU1_ActTMTorque : Outport  Port=2
  MCU1_TMCapacitanceVoltage : Outport  Port=3
  MCU1_ActualTMTorqueValid : Outport  Port=4
  MCU1_MCU1 PrechargeAllow : Outport  Port=5
  MCU1_TMStatus : Outport  Port=6
  MCU1_TMErrorStatus : Outport  Port=7
  MCU1_TM MAMTorque : Outport  Port=8
  MCU1_TM MAGTorque : Outport  Port=9
  MCU1_CalTMTorque : Outport  Port=10
  MCU1_CoolingRequest : Outport  Port=11
  PWM_Status : Outport  Port=12
  EM_trq_req : Outport  Port=13
  bool_MCUPwrDwnAllow : Outport  Port=14
  wires:
  Ground/1 -> MCU1_TMSpeed/1
  Ground1/1 -> MCU1_ActTMTorque/1
  Ground2/1 -> MCU1_TMCapacitanceVoltage/1
  Ground3/1 -> MCU1_ActualTMTorqueValid/1
  Ground4/1 -> MCU1_MCU1 PrechargeAllow/1
  Ground5/1 -> MCU1_TMStatus/1
  Ground6/1 -> MCU1_TMErrorStatus/1
  Ground7/1 -> MCU1_TM MAMTorque/1
  Ground8/1 -> MCU1_TM MAGTorque/1
  Ground9/1 -> MCU1_CalTMTorque/1
  Ground10/1 -> MCU1_CoolingRequest/1
  Ground11/1 -> PWM_Status/1
  In1/1 -> Terminator/1
  Ground12/1 -> EM_trq_req/1
  Constant11/1 -> bool_MCUPwrDwnAllow/1

== system HQEV_MiL_20160830_integrate/MiL/Test_Integration/MCU_RR/MCU/MCU/Subsystem14/Precharge/Subsystem ==
  In1 : Inport
  Bus Selector : BusSelector  OutputSignals=Motor_R.EM2_spd,Motor_R.EM2_U
  Constant{,3..10} (9 alike) : Constant  Value=0
  Constant1 : Constant
  Constant11 : Constant
  Constant2 : Constant
  Unit Delay : UnitDelay  SampleTime=-1
  Unit Delay1 : UnitDelay  SampleTime=-1
  MCU1_TMSpeed : Outport
  MCU1_ActTMTorque : Outport  Port=2
  MCU1_TMCapacitanceVoltage : Outport  Port=3
  MCU1_ActualTMTorqueValid : Outport  Port=4
  MCU1_MCU1 PrechargeAllow : Outport  Port=5
  MCU1_TMStatus : Outport  Port=6
  MCU1_TMErrorStatus : Outport  Port=7
  MCU1_TM MAMTorque : Outport  Port=8
  MCU1_TM MAGTorque : Outport  Port=9
  MCU1_CalTMTorque : Outport  Port=10
  MCU1_CoolingRequest : Outport  Port=11
  PWM_Status : Outport  Port=12
  EM_trq_req : Outport  Port=13
  bool_MCUPwrDwnAllow : Outport  Port=14
  wires:
  Constant7/1 -> MCU1_CoolingRequest/1
  Constant8/1 -> PWM_Status/1
  Constant6/1 -> MCU1_CalTMTorque/1
  Constant10/1 -> MCU1_ActTMTorque/1
  Constant/1 -> MCU1_ActualTMTorqueValid/1
  Constant1/1 -> MCU1_MCU1 PrechargeAllow/1
  Constant2/1 -> MCU1_TMStatus/1
  Constant3/1 -> MCU1_TMErrorStatus/1
  Constant4/1 -> MCU1_TM MAMTorque/1
  Constant5/1 -> MCU1_TM MAGTorque/1
  In1/1 -> Bus Selector/1
  Bus Selector/1 -> Unit Delay/1  "<EM2_spd>"
  Bus Selector/2 -> Unit Delay1/1  "<EM2_U>"
  Unit Delay/1 -> MCU1_TMSpeed/1
  Unit Delay1/1 -> MCU1_TMCapacitanceVoltage/1
  Constant9/1 -> EM_trq_req/1
  Constant11/1 -> bool_MCUPwrDwnAllow/1

== system HQEV_MiL_20160830_integrate/MiL/Test_Integration/MCU_RR/MCU/MCU/Subsystem14/Rapid_Discharge/Subsystem ==
  In1 : Inport
  Bus Selector : BusSelector  OutputSignals=Motor_R.EM2_spd,Motor_R.EM2_U
  Constant{,1..2,4..9} (9 alike) : Constant  Value=0
  Constant11 : Constant
  Constant3 : Constant  Value=6
  Subsystem : Subsystem
  Unit Delay : UnitDelay  SampleTime=-1
  Unit Delay1 : UnitDelay  SampleTime=-1
  MCU1_TMSpeed : Outport
  MCU1_ActTMTorque : Outport  Port=2
  MCU1_TMCapacitanceVoltage : Outport  Port=3
  MCU1_ActualTMTorqueValid : Outport  Port=4
  MCU1_MCU1 PrechargeAllow : Outport  Port=5
  MCU1_TMStatus : Outport  Port=6
  MCU1_TMErrorStatus : Outport  Port=7
  MCU1_TM MAMTorque : Outport  Port=8
  MCU1_TM MAGTorque : Outport  Port=9
  MCU1_CalTMTorque : Outport  Port=10
  MCU1_CoolingRequest : Outport  Port=11
  PWM_Status : Outport  Port=12
  EM_trq_req : Outport  Port=13
  bool_MCUPwrDwnAllow : Outport  Port=14
  wires:
  Constant/1 -> MCU1_ActTMTorque/1
  Constant1/1 -> MCU1_ActualTMTorqueValid/1
  Constant2/1 -> MCU1_MCU1 PrechargeAllow/1
  Constant3/1 -> MCU1_TMStatus/1
  Constant4/1 -> MCU1_TMErrorStatus/1
  Constant5/1 -> MCU1_TM MAMTorque/1
  Constant6/1 -> MCU1_TM MAGTorque/1
  Constant7/1 -> MCU1_CalTMTorque/1
  Constant8/1 -> MCU1_CoolingRequest/1
  Subsystem/1(PWM) -> PWM_Status/1
  In1/1 -> Bus Selector/1
  Bus Selector/1 -> Subsystem/1(EM_spd), Unit Delay/1  "<EM2_spd>"
  Bus Selector/2 -> Unit Delay1/1  "<EM2_U>"
  Unit Delay/1 -> MCU1_TMSpeed/1
  Unit Delay1/1 -> MCU1_TMCapacitanceVoltage/1
  Constant9/1 -> EM_trq_req/1
  Constant11/1 -> bool_MCUPwrDwnAllow/1

== system HQEV_MiL_20160830_integrate/MiL/Test_Integration/MCU_RR/MCU/MCU/Subsystem14/Sleep/Subsystem ==
  In1 : Inport
  Constant : Constant  Value=0
  Constant11 : Constant
  Ground{,1..4,6..12} (12 alike) : Ground
  Terminator : Terminator
  MCU1_TMSpeed : Outport
  MCU1_ActTMTorque : Outport  Port=2
  MCU1_TMCapacitanceVoltage : Outport  Port=3
  MCU1_ActualTMTorqueValid : Outport  Port=4
  MCU1_MCU1 PrechargeAllow : Outport  Port=5
  MCU1_TMStatus : Outport  Port=6
  MCU1_TMErrorStatus : Outport  Port=7
  MCU1_TM MAMTorque : Outport  Port=8
  MCU1_TM MAGTorque : Outport  Port=9
  MCU1_CalTMTorque : Outport  Port=10
  MCU1_CoolingRequest : Outport  Port=11
  PWM_Status : Outport  Port=12
  EM_trq_req : Outport  Port=13
  bool_MCUPwrDwnAllow : Outport  Port=14
  wires:
  Ground/1 -> MCU1_TMSpeed/1
  Ground1/1 -> MCU1_ActTMTorque/1
  Ground2/1 -> MCU1_TMCapacitanceVoltage/1
  Ground3/1 -> MCU1_ActualTMTorqueValid/1
  Ground4/1 -> MCU1_MCU1 PrechargeAllow/1
  Constant/1 -> MCU1_TMStatus/1
  Ground6/1 -> MCU1_TMErrorStatus/1
  Ground7/1 -> MCU1_TM MAMTorque/1
  Ground8/1 -> MCU1_TM MAGTorque/1
  Ground9/1 -> MCU1_CalTMTorque/1
  Ground10/1 -> MCU1_CoolingRequest/1
  Ground11/1 -> PWM_Status/1
  Ground12/1 -> EM_trq_req/1
  In1/1 -> Terminator/1
  Constant11/1 -> bool_MCUPwrDwnAllow/1

== system HQEV_MiL_20160830_integrate/MiL/Test_Integration/MCU_RR/MCU/MCU/Subsystem14/Standby/Subsystem ==
  In1 : Inport
  Bus Selector : BusSelector  OutputSignals=Motor_R.EM2_spd,Motor_R.EM2_U
  Constant{,1,3..7,9..10} (9 alike) : Constant  Value=0
  Constant11 : Constant
  Constant2 : Constant  Value=2
  Subsystem : Subsystem
  Unit Delay : UnitDelay  SampleTime=-1
  Unit Delay1 : UnitDelay  SampleTime=-1
  MCU1_TMSpeed : Outport
  MCU1_ActTMTorque : Outport  Port=2
  MCU1_TMCapacitanceVoltage : Outport  Port=3
  MCU1_ActualTMTorqueValid : Outport  Port=4
  MCU1_MCU1 PrechargeAllow : Outport  Port=5
  MCU1_TMStatus : Outport  Port=6
  MCU1_TMErrorStatus : Outport  Port=7
  MCU1_TM MAMTorque : Outport  Port=8
  MCU1_TM MAGTorque : Outport  Port=9
  MCU1_CalTMTorque : Outport  Port=10
  MCU1_CoolingRequest : Outport  Port=11
  PWM_Status : Outport  Port=12
  EM_trq_req : Outport  Port=13
  bool_MCUPwrDwnAllow : Outport  Port=14
  wires:
  Constant10/1 -> MCU1_ActTMTorque/1
  Constant/1 -> MCU1_ActualTMTorqueValid/1
  Constant1/1 -> MCU1_MCU1 PrechargeAllow/1
  Constant2/1 -> MCU1_TMStatus/1
  Constant3/1 -> MCU1_TMErrorStatus/1
  Constant4/1 -> MCU1_TM MAMTorque/1
  Constant5/1 -> MCU1_TM MAGTorque/1
  Constant6/1 -> MCU1_CalTMTorque/1
  Constant7/1 -> MCU1_CoolingRequest/1
  Subsystem/1(PWM) -> PWM_Status/1
  Constant9/1 -> EM_trq_req/1
  In1/1 -> Bus Selector/1
  Bus Selector/1 -> Subsystem/1(EM_spd), Unit Delay/1  "<EM2_spd>"
  Bus Selector/2 -> Unit Delay1/1  "<EM2_U>"
  Unit Delay/1 -> MCU1_TMSpeed/1
  Unit Delay1/1 -> MCU1_TMCapacitanceVoltage/1
  Constant11/1 -> bool_MCUPwrDwnAllow/1

== system HQEV_MiL_20160830_integrate/MiL/Test_Integration/MCU_RR/MCU/MCU/Subsystem14/Stop/Subsystem ==
  In1 : Inport
  Bus Selector : BusSelector  OutputSignals=Motor_R.EM2_spd,Motor_R.EM2_U
  Constant{,3..7,9..10} (8 alike) : Constant  Value=0
  Constant1 : Constant
  Constant11 : Constant
  Constant2 : Constant  Value=4
  Data Type Conversion : DataTypeConversion
  Data Type Conversion1 : DataTypeConversion
  Subsystem : Subsystem
  MCU1_TMSpeed : Outport
  MCU1_ActTMTorque : Outport  Port=2
  MCU1_TMCapacitanceVoltage : Outport  Port=3
  MCU1_ActualTMTorqueValid : Outport  Port=4
  MCU1_MCU1 PrechargeAllow : Outport  Port=5
  MCU1_TMStatus : Outport  Port=6
  MCU1_TMErrorStatus : Outport  Port=7
  MCU1_TM MAMTorque : Outport  Port=8
  MCU1_TM MAGTorque : Outport  Port=9
  MCU1_CalTMTorque : Outport  Port=10
  MCU1_CoolingRequest : Outport  Port=11
  PWM_Status : Outport  Port=12
  EM_trq_req : Outport  Port=13
  bool_MCUPwrDwnAllow : Outport  Port=14
  wires:
  Constant10/1 -> MCU1_ActTMTorque/1
  Constant/1 -> MCU1_ActualTMTorqueValid/1
  Constant1/1 -> MCU1_MCU1 PrechargeAllow/1
  Constant2/1 -> MCU1_TMStatus/1
  Constant3/1 -> MCU1_TMErrorStatus/1
  Constant4/1 -> MCU1_TM MAMTorque/1
  Constant5/1 -> MCU1_TM MAGTorque/1
  Constant6/1 -> MCU1_CalTMTorque/1
  Constant7/1 -> MCU1_CoolingRequest/1
  Constant9/1 -> EM_trq_req/1
  Subsystem/1(PWM) -> PWM_Status/1
  Bus Selector/1 -> Subsystem/1(EM_spd), Data Type Conversion/1  "<EM2_spd>"
  In1/1 -> Bus Selector/1
  Bus Selector/2 -> Data Type Conversion1/1  "<EM2_U>"
  Data Type Conversion/1 -> MCU1_TMSpeed/1
  Data Type Conversion1/1 -> MCU1_TMCapacitanceVoltage/1
  Constant11/1 -> bool_MCUPwrDwnAllow/1

== system HQEV_MiL_20160830_integrate/MiL/Test_Integration/MCU_RR/MCU/MCU/Subsystem14/Torque_Control/Subsystem ==
  In1 : Inport
  Bus Selector : BusSelector  OutputSignals=Motor_R.EM2_spd,Motor_R.EM2_trq_out,Motor_R.EM2_U,HCU.HCU_TMTorqueRequestToMCU2
  Constant : Constant
  Constant1 : Constant
  Constant11 : Constant  Value=0
  Constant2 : Constant  Value=3
  Constant3 : Constant  Value=0
  Constant4 : Constant  Value=0
  Constant5 : Constant
  Constant6 : Constant  Value=300
  Data Type Conversion2 : DataTypeConversion
  Max_Torque : Subsystem  TreatAsAtomicUnit=on
  Unit Delay{,1..4} (5 alike) : UnitDelay  SampleTime=-1
  MCU1_TMSpeed : Outport
  MCU1_ActTMTorque : Outport  Port=2
  MCU1_TMCapacitanceVoltage : Outport  Port=3
  MCU1_ActualTMTorqueValid : Outport  Port=4
  MCU1_MCU1 PrechargeAllow : Outport  Port=5
  MCU1_TMStatus : Outport  Port=6
  MCU1_TMErrorStatus : Outport  Port=7
  MCU1_TM MAMTorque : Outport  Port=8
  MCU1_TM MAGTorque : Outport  Port=9
  MCU1_CalTMTorque : Outport  Port=10
  MCU1_CoolingRequest : Outport  Port=11
  PWM_Status : Outport  Port=12
  EM_trq_req : Outport  Port=13
  bool_MCUPwrDwnAllow : Outport  Port=14
  wires:
  Max_Torque/1(Max_Mot_Torque) -> MCU1_TM MAMTorque/1
  Max_Torque/2(Max_Gen_Torque) -> MCU1_TM MAGTorque/1
  Constant/1 -> MCU1_ActualTMTorqueValid/1
  Constant1/1 -> MCU1_MCU1 PrechargeAllow/1
  Constant2/1 -> MCU1_TMStatus/1
  Constant3/1 -> MCU1_TMErrorStatus/1
  Constant4/1 -> MCU1_CoolingRequest/1
  Constant5/1 -> PWM_Status/1
  In1/1 -> Bus Selector/1
  Bus Selector/1 -> Max_Torque/2(EM_spd), Unit Delay/1  "<EM2_spd>"
  Bus Selector/2 -> Unit Delay1/1, Unit Delay4/1  "<EM2_trq_out>"
  Bus Selector/3 -> Unit Delay2/1  "<EM2_U>"
  Constant6/1 -> Max_Torque/1(EM_Volt)
  Bus Selector/4 -> Unit Delay3/1  "<HCU_TMTorqueRequestToMCU2>"
  Unit Delay/1 -> MCU1_TMSpeed/1
  Unit Delay1/1 -> MCU1_ActTMTorque/1
  Unit Delay2/1 -> MCU1_TMCapacitanceVoltage/1
  Unit Delay3/1 -> Data Type Conversion2/1
  Unit Delay4/1 -> MCU1_CalTMTorque/1
  Data Type Conversion2/1 -> EM_trq_req/1
  Constant11/1 -> bool_MCUPwrDwnAllow/1

== system HQEV_MiL_20160830_integrate/MiL/Test_Integration/Motor_FF/Motor/Motor/eMotor/Electric Power/Motor Electric Power ==
  In1 : Inport
  Bus Selector1 : BusSelector  OutputSignals=P_Mech,eta
  Bus Selector2 : BusSelector  OutputSignals=P_Mech
  Bus Selector3 : BusSelector  OutputSignals=P_Mech,eta
  Bus Selector4 : BusSelector  OutputSignals=T_Mot,n_Mot
  Divide : Product  Inputs=*/
  Divide1 : Product  Inputs=**
  Divide2 : Product  Inputs=**
  Subtract : Sum  Inputs=+-
  Switch : Switch  Criteria=u2 > Threshold
  abs : Subsystem
  abs1 : Subsystem
  abs2 : Subsystem
  EM1_pwr_elec : Outport
  EM1_pwr_loss : Outport  Port=2
  wires:
  Divide/1 -> Switch/1
  Divide1/1 -> Switch/3
  Bus Selector1/1 -> Divide/1  "<P_Mech>"
  Bus Selector1/2 -> Divide/2  "<eta>"
  Bus Selector3/1 -> Divide1/1  "<P_Mech>"
  Bus Selector3/2 -> Divide1/2  "<eta>"
  Switch/1 -> EM1_pwr_elec/1, abs/1(In1)
  In1/1 -> Bus Selector1/1, Bus Selector4/1, Bus Selector3/1, Bus Selector2/1
  Bus Selector2/1 -> abs1/1(In1)  "<P_Mech>"
  abs1/1(Out1) -> Subtract/2
  Bus Selector4/1 -> Divide2/1  "<T_Mot>"
  Bus Selector4/2 -> Divide2/2  "<n_Mot>"
  Divide2/1 -> Switch/2
  abs/1(Out1) -> Subtract/1
  Subtract/1 -> abs2/1(In1)
  abs2/1(Out1) -> EM1_pwr_loss/1

== system HQEV_MiL_20160830_integrate/MiL/Test_Integration/Motor_FF/Motor/Motor/eMotor/Electric Power/Motor Mechanical Power ==
  In1 : Inport
  Bus Selector2 : BusSelector  OutputSignals=n_Mot,T_Mot
  Constant : Constant  Value=9550
  Constant1 : Constant  Value=1000
  Divide2 : Product  Inputs=*/
  Product : Product  RndMeth=Zero
  Product1 : Product  RndMeth=Zero
  EM_pwr_mech : Outport
  wires:
  Bus Selector2/1 -> Product/1  "<n_Mot>"
  Bus Selector2/2 -> Product/2  "<T_Mot>"
  Product/1 -> Divide2/1
  Constant/1 -> Divide2/2
  In1/1 -> Bus Selector2/1
  Divide2/1 -> Product1/1
  Constant1/1 -> Product1/2
  Product1/1 -> EM_pwr_mech/1

== system HQEV_MiL_20160830_integrate/MiL/Test_Integration/Motor_RR/Motor/Motor1/eMotor/Electric Power/Motor Electric Power ==
  In1 : Inport
  Bus Selector1 : BusSelector  OutputSignals=P_Mech,eta
  Bus Selector2 : BusSelector  OutputSignals=P_Mech
  Bus Selector3 : BusSelector  OutputSignals=P_Mech,eta
  Bus Selector4 : BusSelector  OutputSignals=T_Mot,n_Mot
  Divide : Product  Inputs=*/
  Divide1 : Product  Inputs=**
  Divide2 : Product  Inputs=**
  Subtract : Sum  Inputs=+-
  Switch : Switch  Criteria=u2 > Threshold
  abs : Subsystem
  abs1 : Subsystem
  abs2 : Subsystem
  EM1_pwr_elec : Outport
  EM1_pwr_loss : Outport  Port=2
  wires:
  Divide/1 -> Switch/1
  Divide1/1 -> Switch/3
  Bus Selector1/1 -> Divide/1  "<P_Mech>"
  Bus Selector1/2 -> Divide/2  "<eta>"
  Bus Selector3/1 -> Divide1/1  "<P_Mech>"
  Bus Selector3/2 -> Divide1/2  "<eta>"
  Switch/1 -> EM1_pwr_elec/1, abs/1(In1)
  In1/1 -> Bus Selector1/1, Bus Selector4/1, Bus Selector3/1, Bus Selector2/1
  Bus Selector2/1 -> abs1/1(In1)  "<P_Mech>"
  abs1/1(Out1) -> Subtract/2
  Bus Selector4/1 -> Divide2/1  "<T_Mot>"
  Bus Selector4/2 -> Divide2/2  "<n_Mot>"
  Divide2/1 -> Switch/2
  abs/1(Out1) -> Subtract/1
  Subtract/1 -> abs2/1(In1)
  abs2/1(Out1) -> EM1_pwr_loss/1

== system HQEV_MiL_20160830_integrate/MiL/Test_Integration/Motor_RR/Motor/Motor1/eMotor/Electric Power/Motor Mechanical Power ==
  In1 : Inport
  Bus Selector2 : BusSelector  OutputSignals=n_Mot,T_Mot
  Constant : Constant  Value=9550
  Constant1 : Constant  Value=1000
  Divide2 : Product  Inputs=*/
  Product : Product  RndMeth=Zero
  Product1 : Product  RndMeth=Zero
  EM_pwr_mech : Outport
  wires:
  Bus Selector2/1 -> Product/1  "<n_Mot>"
  Bus Selector2/2 -> Product/2  "<T_Mot>"
  Product/1 -> Divide2/1
  Constant/1 -> Divide2/2
  In1/1 -> Bus Selector2/1
  Divide2/1 -> Product1/1
  Constant1/1 -> Product1/2
  Product1/1 -> EM_pwr_mech/1

== system HQEV_MiL_20160830_integrate/MiL/Test_Integration/Reducer_F/FinalDrive/FinalDrive/Subsystem/Backward/Efficiency ==
  T_in : Inport
  "Temp " : Inport  Port=2
  "Omega_in " : Inport  Port=3
  Terminator : Terminator
  Terminator1 : Terminator
  Terminator2 : Terminator
  eta_constant : Constant  Value=0.94
  eta : Outport
  wires:
  eta_constant/1 -> eta/1
  "Omega_in "/1 -> Terminator/1
  T_in/1 -> Terminator1/1
  "Temp "/1 -> Terminator2/1

== system HQEV_MiL_20160830_integrate/MiL/Test_Integration/Reducer_F/FinalDrive/FinalDrive/Subsystem/Forward/Efficiency ==
  T_in : Inport
  "Temp " : Inport  Port=2
  "Omega_in " : Inport  Port=3
  Terminator : Terminator
  Terminator1 : Terminator
  Terminator2 : Terminator
  eta_constant : Constant  Value=0.94
  eta : Outport
  wires:
  eta_constant/1 -> eta/1
  "Omega_in "/1 -> Terminator/1
  T_in/1 -> Terminator1/1
  "Temp "/1 -> Terminator2/1

== system HQEV_MiL_20160830_integrate/MiL/Test_Integration/Reducer_R/FinalDrive/FinalDrive/Subsystem/Backward/Efficiency ==
  T_in : Inport
  "Temp " : Inport  Port=2
  "Omega_in " : Inport  Port=3
  Terminator : Terminator
  Terminator1 : Terminator
  Terminator2 : Terminator
  eta_constant : Constant  Value=0.94
  eta : Outport
  wires:
  "Temp "/1 -> Terminator2/1
  T_in/1 -> Terminator1/1
  "Omega_in "/1 -> Terminator/1
  eta_constant/1 -> eta/1

== system HQEV_MiL_20160830_integrate/MiL/Test_Integration/Reducer_R/FinalDrive/FinalDrive/Subsystem/Forward/Efficiency ==
  T_in : Inport
  "Temp " : Inport  Port=2
  "Omega_in " : Inport  Port=3
  Terminator : Terminator
  Terminator1 : Terminator
  Terminator2 : Terminator
  eta_constant : Constant  Value=0.94
  eta : Outport
  wires:
  "Temp "/1 -> Terminator2/1
  T_in/1 -> Terminator1/1
  "Omega_in "/1 -> Terminator/1
  eta_constant/1 -> eta/1
